simulink model "s_r_p_i"  (R2026a)
settings: Solver=VariableStepAuto
libraries: simulink x1
settings Model: Creator=tanmay  LastModifiedBy=tanmay

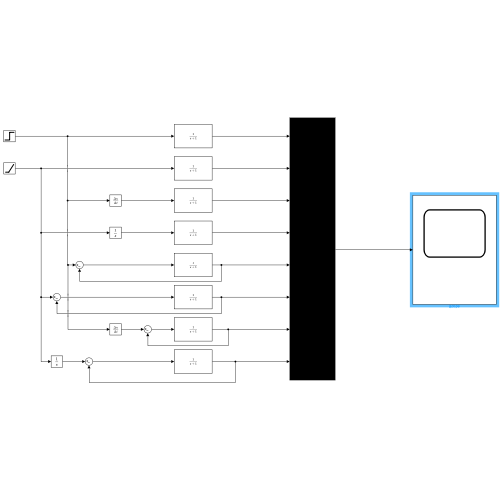
[thumbnail: Simulink's stored preview of the top-level diagram]
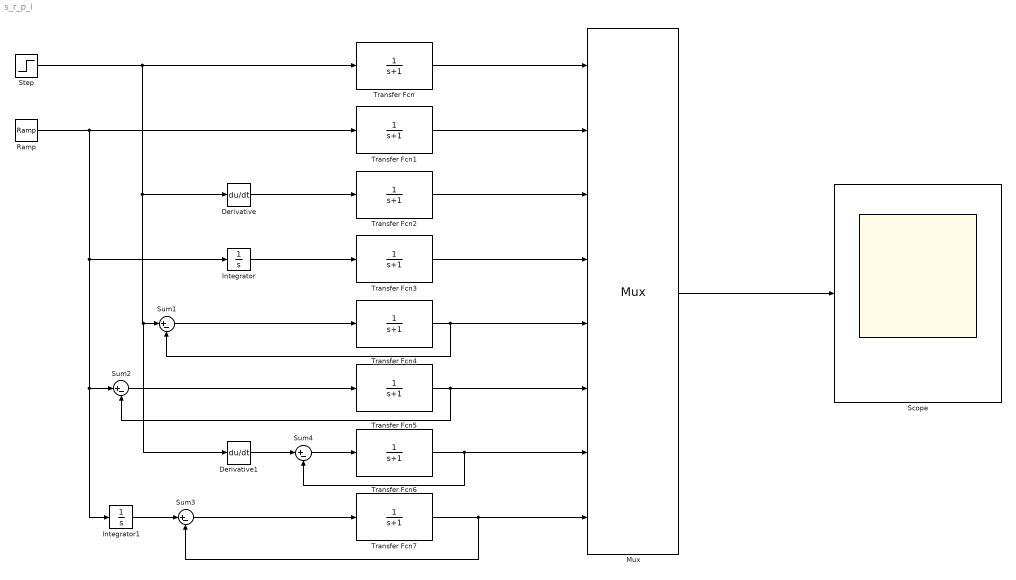
== system s_r_p_i ==
  Derivative : Derivative
  Derivative1 : Derivative
  Integrator : Integrator
  Integrator1 : Integrator
  Mux : Mux  Inputs=8
  Ramp : simulink/Sources/Ramp  slope=1  start=0  InitialOutput=0
  Scope : Scope
      settings: ActiveDisplayYMinimum=-5.1249943250027234  ActiveDisplayYMaximum=46.124948925024519
  Step : Step  SampleTime=0
  Sum{1..4} (4 alike) : Sum  Inputs=|+-
  Transfer Fcn{,1..7} (8 alike) : TransferFcn  Denominator=[1 1]
  wires:
  Mux/1 -> Scope/1
  Step/1 -> Derivative1/1, Sum1/1, Derivative/1, Transfer Fcn/1
  Derivative/1 -> Transfer Fcn2/1
  Integrator/1 -> Transfer Fcn3/1
  Ramp/1 -> Integrator1/1, Sum2/1, Integrator/1, Transfer Fcn1/1
  Sum1/1 -> Transfer Fcn4/1
  Transfer Fcn4/1 -> Mux/5, Sum1/2
  Transfer Fcn3/1 -> Mux/4
  Transfer Fcn2/1 -> Mux/3
  Transfer Fcn1/1 -> Mux/2
  Transfer Fcn/1 -> Mux/1
  Sum2/1 -> Transfer Fcn5/1
  Transfer Fcn5/1 -> Mux/6, Sum2/2
  Transfer Fcn6/1 -> Sum4/2, Mux/7
  Sum4/1 -> Transfer Fcn6/1
  Derivative1/1 -> Sum4/1
  Integrator1/1 -> Sum3/1
  Sum3/1 -> Transfer Fcn7/1
  Transfer Fcn7/1 -> Sum3/2, Mux/8
